simulink model "Smart_City_QCar2_VIRTUAL_car5_r2020a"  (R2020a)
settings: Solver=ode1  StartTime=0.0  StopTime=inf  FixedStep=Controller_Sample_Time  RelTol=1e-3  EnableMultiTasking=on
undefined symbols (not defined in the file): Audio_Sample_Time, cameraStepSize, CSI_Sample_Time, DiscIntNeverNeededParam, gcbh, ImageDisplay_Sample_Time, Initialization_Time, Joystick_Sample_Time, JPEG, LiDAR_Sample_Time, map_mask, NN_Sample_Time, path_x, path_x2, path_x3, path_x4, path_x5, path_x6, path_x7, path_y, path_y2, path_y3, path_y4, path_y5, path_y6, path_y7, qc_get_step_size, RealSense_Sample_Time, video_display_show
libraries: quarc_library x61, simulink_extras x9, simulink x5
(part 3 of 4)

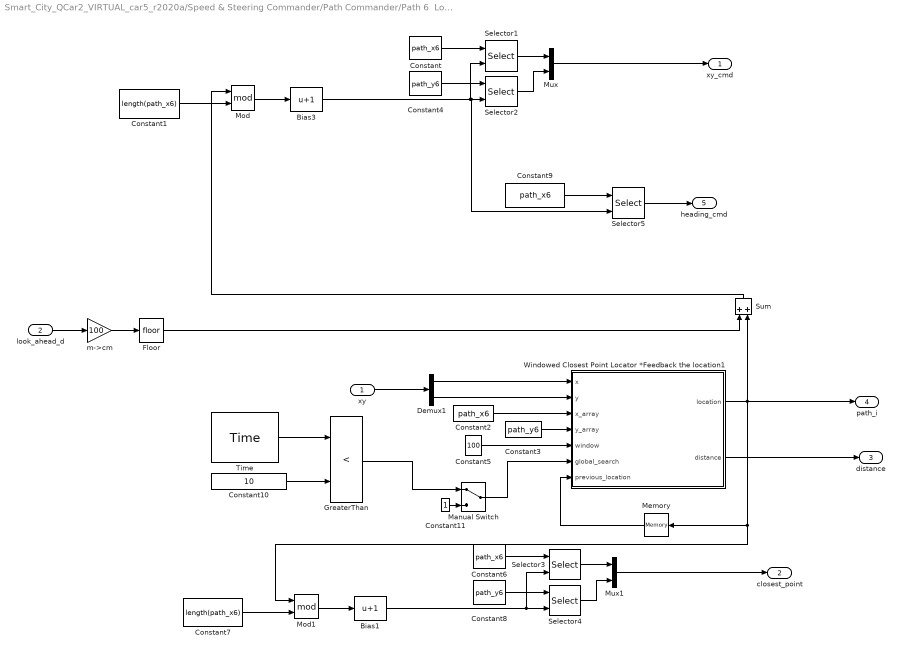
== system Smart_City_QCar2_VIRTUAL_car5_r2020a/Speed & Steering Commander/Path Commander/Path 6  Look Ahead Generator ==
  xy : Inport
  look_ahead_d : Inport  Port=2
  Bias1 : Bias  Bias=1
  Bias3 : Bias  Bias=1
  Constant{,2,6,9} (4 alike) : Constant  Value=path_x6
  Constant1 : Constant  Value=length(path_x6)
  Constant10 : Constant  Value=10
  Constant11 : Constant
  Constant3 : Constant  Value=path_y6
  Constant4 : Constant  Value=path_y6
  Constant5 : Constant  Value=100
  Constant7 : Constant  Value=length(path_x6)
  Constant8 : Constant  Value=path_y6
  Demux1 : Demux  Outputs=2
  Floor : Rounding
  GreaterThan : RelationalOperator  Operator=<  OutDataTypeStr=boolean  RndMeth=Simplest
  Manual Switch : ManualSwitch
  Memory : Memory  InitialCondition=1  InheritSampleTime=on  LinearizeMemory=on  LinearizeAsDelay=on
  Mod : Math  Operator=mod  SaturateOnIntegerOverflow=on
  Mod1 : Math  Operator=mod  SaturateOnIntegerOverflow=on
  Mux : Mux  Inputs=2
  Mux1 : Mux  Inputs=2
  Selector{1..5} (5 alike) : Selector  InputPortWidth=length(path_x6)  IndexOptions=Index vector (port)  Indices=[1 3]  OutputSizes=1
  Sum : Sum
  Time : quarc_library/Sources/Time/Time  time_source=Wall clock  sample_time=qc_get_step_size
  Windowed Closest Point Locator *Feedback the location1 : MATLAB Function  TreatAsAtomicUnit=on
  m->cm : Gain  Gain=100
  xy_cmd : Outport
  closest_point : Outport  Port=2
  distance : Outport  Port=3
  path_i : Outport  Port=4
  heading_cmd : Outport  Port=5
  wires:
  Windowed Closest Point Locator *Feedback the location1/1(location) -> Mod1/1, Memory/1, path_i/1, Sum/2
  Memory/1 -> Windowed Closest Point Locator *Feedback the location1/7(previous_location)
  Constant5/1 -> Windowed Closest Point Locator *Feedback the location1/5(window)
  Selector5/1 -> heading_cmd/1
  Constant9/1 -> Selector5/1
  Bias3/1 -> Selector2/2, Selector5/2, Selector1/2
  Windowed Closest Point Locator *Feedback the location1/2(distance) -> distance/1
  Selector2/1 -> Mux/2
  Mux/1 -> xy_cmd/1
  Constant4/1 -> Selector2/1
  Selector1/1 -> Mux/1
  Constant/1 -> Selector1/1
  Floor/1 -> Sum/1
  m->cm/1 -> Floor/1
  look_ahead_d/1 -> m->cm/1
  xy/1 -> Demux1/1
  Mod/1 -> Bias3/1
  Demux1/2 -> Windowed Closest Point Locator *Feedback the location1/2(y)
  Sum/1 -> Mod/1
  Constant1/1 -> Mod/2
  Constant3/1 -> Windowed Closest Point Locator *Feedback the location1/4(y_array)
  Constant2/1 -> Windowed Closest Point Locator *Feedback the location1/3(x_array)
  Demux1/1 -> Windowed Closest Point Locator *Feedback the location1/1(x)
  Mux1/1 -> closest_point/1
  Mod1/1 -> Bias1/1
  Selector4/1 -> Mux1/2
  Constant7/1 -> Mod1/2
  Selector3/1 -> Mux1/1
  Constant8/1 -> Selector4/1
  Bias1/1 -> Selector3/2, Selector4/2
  Constant6/1 -> Selector3/1
  Time/1 -> GreaterThan/1
  Constant10/1 -> GreaterThan/2
  Manual Switch/1 -> Windowed Closest Point Locator *Feedback the location1/6(global_search)
  Constant11/1 -> Manual Switch/2
  GreaterThan/1 -> Manual Switch/1

== system Smart_City_QCar2_VIRTUAL_car5_r2020a/Speed & Steering Commander/Path Commander/Path 7  Look Ahead Generator ==
  xy : Inport
  look_ahead_d : Inport  Port=2
  Bias1 : Bias  Bias=1
  Bias3 : Bias  Bias=1
  Constant{,2,6,9} (4 alike) : Constant  Value=path_x7
  Constant1 : Constant  Value=length(path_x7)
  Constant10 : Constant  Value=10
  Constant11 : Constant
  Constant3 : Constant  Value=path_y7
  Constant4 : Constant  Value=path_y7
  Constant5 : Constant  Value=100
  Constant7 : Constant  Value=length(path_x7)
  Constant8 : Constant  Value=path_y7
  Demux1 : Demux  Outputs=2
  Floor : Rounding
  GreaterThan : RelationalOperator  Operator=<  OutDataTypeStr=boolean  RndMeth=Simplest
  Manual Switch : ManualSwitch
  Memory : Memory  InitialCondition=1  InheritSampleTime=on  LinearizeMemory=on  LinearizeAsDelay=on
  Mod : Math  Operator=mod  SaturateOnIntegerOverflow=on
  Mod1 : Math  Operator=mod  SaturateOnIntegerOverflow=on
  Mux : Mux  Inputs=2
  Mux1 : Mux  Inputs=2
  Selector{1..5} (5 alike) : Selector  InputPortWidth=length(path_x7)  IndexOptions=Index vector (port)  Indices=[1 3]  OutputSizes=1
  Sum : Sum
  Time : quarc_library/Sources/Time/Time  time_source=Wall clock  sample_time=qc_get_step_size
  Windowed Closest Point Locator *Feedback the location1 : MATLAB Function  TreatAsAtomicUnit=on
  m->cm : Gain  Gain=100
  xy_cmd : Outport
  closest_point : Outport  Port=2
  distance : Outport  Port=3
  path_i : Outport  Port=4
  heading_cmd : Outport  Port=5
  wires:
  Windowed Closest Point Locator *Feedback the location1/1(location) -> Mod1/1, Memory/1, path_i/1, Sum/2
  Memory/1 -> Windowed Closest Point Locator *Feedback the location1/7(previous_location)
  Constant5/1 -> Windowed Closest Point Locator *Feedback the location1/5(window)
  Selector5/1 -> heading_cmd/1
  Constant9/1 -> Selector5/1
  Bias3/1 -> Selector2/2, Selector5/2, Selector1/2
  Windowed Closest Point Locator *Feedback the location1/2(distance) -> distance/1
  Selector2/1 -> Mux/2
  Mux/1 -> xy_cmd/1
  Constant4/1 -> Selector2/1
  Selector1/1 -> Mux/1
  Constant/1 -> Selector1/1
  Floor/1 -> Sum/1
  m->cm/1 -> Floor/1
  look_ahead_d/1 -> m->cm/1
  xy/1 -> Demux1/1
  Mod/1 -> Bias3/1
  Demux1/2 -> Windowed Closest Point Locator *Feedback the location1/2(y)
  Sum/1 -> Mod/1
  Constant1/1 -> Mod/2
  Constant3/1 -> Windowed Closest Point Locator *Feedback the location1/4(y_array)
  Constant2/1 -> Windowed Closest Point Locator *Feedback the location1/3(x_array)
  Demux1/1 -> Windowed Closest Point Locator *Feedback the location1/1(x)
  Mux1/1 -> closest_point/1
  Mod1/1 -> Bias1/1
  Selector4/1 -> Mux1/2
  Constant7/1 -> Mod1/2
  Selector3/1 -> Mux1/1
  Constant8/1 -> Selector4/1
  Bias1/1 -> Selector3/2, Selector4/2
  Constant6/1 -> Selector3/1
  Time/1 -> GreaterThan/1
  Constant10/1 -> GreaterThan/2
  Manual Switch/1 -> Windowed Closest Point Locator *Feedback the location1/6(global_search)
  Constant11/1 -> Manual Switch/2
  GreaterThan/1 -> Manual Switch/1

== system Smart_City_QCar2_VIRTUAL_car5_r2020a/Speed & Steering Commander/Steering Based on LiDAR/Direction Vector Generator ==
  xy_command : Inport
  xy : Inport  Port=2
  heading : Inport  Port=3
  Demux : Demux  Outputs=2
  Display2 : Display  Commented=on
      settings: Decimation=100
  Display5 : Display  Commented=on
      settings: Decimation=100
  Display8 : Display  Commented=on
      settings: Decimation=100
  Radians to Degrees1 : simulink_extras/Transformations/Radians to Degrees
  Radians to Degrees3 : simulink_extras/Transformations/Radians to Degrees
  Signed Sqrt : Sqrt  SaturateOnIntegerOverflow=on
  Square : Math  Operator=square  SaturateOnIntegerOverflow=on
  Sum : Sum  Inputs=+-
  Sum1 : Sum  Inputs=+
  Sum3 : Sum  Inputs=+-
  Trigonometric Function : Trigonometry  Operator=atan2
  distance : Outport
  aoa : Outport  Port=2
  wires:
  heading/1 -> Sum3/2
  Sum/1 -> Demux/1, Square/1
  Radians to Degrees3/1 -> Display2/1
  Radians to Degrees1/1 -> Display5/1
  Demux/2 -> Trigonometric Function/1
  Sum1/1 -> Signed Sqrt/1
  Sum3/1 -> aoa/1, Radians to Degrees3/1
  xy/1 -> Sum/2
  Signed Sqrt/1 -> distance/1, Display8/1
  Square/1 -> Sum1/1
  Trigonometric Function/1 -> Radians to Degrees1/1, Sum3/1
  Demux/1 -> Trigonometric Function/2
  xy_command/1 -> Sum/1

== system Smart_City_QCar2_VIRTUAL_car5_r2020a/Speed & Steering Commander/Traffic Zone 1/Greater Than Threshold ==
  Signal : Inport
  Threshold : Inport  Port=2
  Duration : Inport  Port=3
  Data Type Conversion : DataTypeConversion
  Discrete-Time Integrator : DiscreteIntegrator  Priority=1  ExternalReset=level  SampleTime=qc_get_step_size  ICPrevOutput=DiscIntNeverNeededParam  ICPrevScaledInput=DiscIntNeverNeededParam
  Logical Operator : Logic  Operator=NOT  AllPortsSameDT=off  OutDataTypeStr=boolean
  Relational Operator : RelationalOperator  RndMeth=Nearest
  Relational Operator1 : RelationalOperator  RndMeth=Nearest
  elapsed : Outport  VectorParamsAs1DForOutWhenUnconnected=off
  time : Outport  Port=2  VectorParamsAs1DForOutWhenUnconnected=off
  wires:
  Data Type Conversion/1 -> Discrete-Time Integrator/1
  Signal/1 -> Relational Operator/1
  Threshold/1 -> Relational Operator/2
  Relational Operator/1 -> Data Type Conversion/1, Logical Operator/1
  Logical Operator/1 -> Discrete-Time Integrator/2
  Discrete-Time Integrator/1 -> Relational Operator1/1, time/1
  Duration/1 -> Relational Operator1/2
  Relational Operator1/1 -> elapsed/1

== system Smart_City_QCar2_VIRTUAL_car5_r2020a/Speed & Steering Commander/Traffic Zone 1/Less Than Threshold ==
  Signal : Inport
  Threshold : Inport  Port=2
  Duration : Inport  Port=3
  Data Type Conversion : DataTypeConversion
  Discrete-Time Integrator : DiscreteIntegrator  Priority=1  ExternalReset=level  SampleTime=qc_get_step_size  ICPrevOutput=DiscIntNeverNeededParam  ICPrevScaledInput=DiscIntNeverNeededParam
  Logical Operator : Logic  Operator=NOT  AllPortsSameDT=off  OutDataTypeStr=boolean
  Relational Operator : RelationalOperator  Operator=<  RndMeth=Nearest
  Relational Operator1 : RelationalOperator  RndMeth=Nearest
  elapsed : Outport  VectorParamsAs1DForOutWhenUnconnected=off
  time : Outport  Port=2  VectorParamsAs1DForOutWhenUnconnected=off
  wires:
  Relational Operator1/1 -> elapsed/1
  Duration/1 -> Relational Operator1/2
  Discrete-Time Integrator/1 -> time/1, Relational Operator1/1
  Logical Operator/1 -> Discrete-Time Integrator/2
  Relational Operator/1 -> Logical Operator/1, Data Type Conversion/1
  Threshold/1 -> Relational Operator/2
  Signal/1 -> Relational Operator/1
  Data Type Conversion/1 -> Discrete-Time Integrator/1

== system Smart_City_QCar2_VIRTUAL_car5_r2020a/Speed & Steering Commander/Traffic Zone 2/Greater Than Threshold ==
  Signal : Inport
  Threshold : Inport  Port=2
  Duration : Inport  Port=3
  Data Type Conversion : DataTypeConversion
  Discrete-Time Integrator : DiscreteIntegrator  Priority=1  ExternalReset=level  SampleTime=qc_get_step_size  ICPrevOutput=DiscIntNeverNeededParam  ICPrevScaledInput=DiscIntNeverNeededParam
  Logical Operator : Logic  Operator=NOT  AllPortsSameDT=off  OutDataTypeStr=boolean
  Relational Operator : RelationalOperator  RndMeth=Nearest
  Relational Operator1 : RelationalOperator  RndMeth=Nearest
  elapsed : Outport  VectorParamsAs1DForOutWhenUnconnected=off
  time : Outport  Port=2  VectorParamsAs1DForOutWhenUnconnected=off
  wires:
  Relational Operator1/1 -> elapsed/1
  Duration/1 -> Relational Operator1/2
  Discrete-Time Integrator/1 -> time/1, Relational Operator1/1
  Logical Operator/1 -> Discrete-Time Integrator/2
  Relational Operator/1 -> Logical Operator/1, Data Type Conversion/1
  Threshold/1 -> Relational Operator/2
  Signal/1 -> Relational Operator/1
  Data Type Conversion/1 -> Discrete-Time Integrator/1

== system Smart_City_QCar2_VIRTUAL_car5_r2020a/Speed & Steering Commander/Traffic Zone 2/Less Than Threshold ==
  Signal : Inport
  Threshold : Inport  Port=2
  Duration : Inport  Port=3
  Data Type Conversion : DataTypeConversion
  Discrete-Time Integrator : DiscreteIntegrator  Priority=1  ExternalReset=level  SampleTime=qc_get_step_size  ICPrevOutput=DiscIntNeverNeededParam  ICPrevScaledInput=DiscIntNeverNeededParam
  Logical Operator : Logic  Operator=NOT  AllPortsSameDT=off  OutDataTypeStr=boolean
  Relational Operator : RelationalOperator  Operator=<  RndMeth=Nearest
  Relational Operator1 : RelationalOperator  RndMeth=Nearest
  elapsed : Outport  VectorParamsAs1DForOutWhenUnconnected=off
  time : Outport  Port=2  VectorParamsAs1DForOutWhenUnconnected=off
  wires:
  Data Type Conversion/1 -> Discrete-Time Integrator/1
  Signal/1 -> Relational Operator/1
  Threshold/1 -> Relational Operator/2
  Relational Operator/1 -> Data Type Conversion/1, Logical Operator/1
  Logical Operator/1 -> Discrete-Time Integrator/2
  Discrete-Time Integrator/1 -> Relational Operator1/1, time/1
  Duration/1 -> Relational Operator1/2
  Relational Operator1/1 -> elapsed/1

== system Smart_City_QCar2_VIRTUAL_car5_r2020a/QCar/Virtual QCar/LED Logic/Greater Than Threshold1 ==
  Signal : Inport
  Threshold : Inport  Port=2
  Duration : Inport  Port=3
  Data Type Conversion : DataTypeConversion
  Discrete-Time Integrator : DiscreteIntegrator  Priority=1  ExternalReset=level  SampleTime=qc_get_step_size  ICPrevOutput=DiscIntNeverNeededParam  ICPrevScaledInput=DiscIntNeverNeededParam
  Logical Operator : Logic  Operator=NOT  AllPortsSameDT=off  OutDataTypeStr=boolean
  Relational Operator : RelationalOperator  RndMeth=Nearest
  Relational Operator1 : RelationalOperator  RndMeth=Nearest
  elapsed : Outport  VectorParamsAs1DForOutWhenUnconnected=off
  time : Outport  Port=2  VectorParamsAs1DForOutWhenUnconnected=off
  wires:
  Data Type Conversion/1 -> Discrete-Time Integrator/1
  Signal/1 -> Relational Operator/1
  Threshold/1 -> Relational Operator/2
  Relational Operator/1 -> Data Type Conversion/1, Logical Operator/1
  Logical Operator/1 -> Discrete-Time Integrator/2
  Discrete-Time Integrator/1 -> Relational Operator1/1, time/1
  Duration/1 -> Relational Operator1/2
  Relational Operator1/1 -> elapsed/1

== system Smart_City_QCar2_VIRTUAL_car5_r2020a/QCar/Virtual QCar/LED Logic/Left Threshold ==
  Signal : Inport
  Threshold : Inport  Port=2
  Duration : Inport  Port=3
  Data Type Conversion : DataTypeConversion
  Discrete-Time Integrator : DiscreteIntegrator  Priority=1  ExternalReset=level  SampleTime=qc_get_step_size  ICPrevOutput=DiscIntNeverNeededParam  ICPrevScaledInput=DiscIntNeverNeededParam
  Logical Operator : Logic  Operator=NOT  AllPortsSameDT=off  OutDataTypeStr=boolean
  Relational Operator : RelationalOperator  RndMeth=Nearest
  Relational Operator1 : RelationalOperator  RndMeth=Nearest
  elapsed : Outport  VectorParamsAs1DForOutWhenUnconnected=off
  time : Outport  Port=2  VectorParamsAs1DForOutWhenUnconnected=off
  wires:
  Data Type Conversion/1 -> Discrete-Time Integrator/1
  Signal/1 -> Relational Operator/1
  Threshold/1 -> Relational Operator/2
  Relational Operator/1 -> Data Type Conversion/1, Logical Operator/1
  Logical Operator/1 -> Discrete-Time Integrator/2
  Discrete-Time Integrator/1 -> Relational Operator1/1, time/1
  Duration/1 -> Relational Operator1/2
  Relational Operator1/1 -> elapsed/1

== system Smart_City_QCar2_VIRTUAL_car5_r2020a/QCar/Virtual QCar/LED Logic/Less Than Threshold1 ==
  Signal : Inport
  Threshold : Inport  Port=2
  Duration : Inport  Port=3
  Data Type Conversion : DataTypeConversion
  Discrete-Time Integrator : DiscreteIntegrator  Priority=1  ExternalReset=level  SampleTime=qc_get_step_size  ICPrevOutput=DiscIntNeverNeededParam  ICPrevScaledInput=DiscIntNeverNeededParam
  Logical Operator : Logic  Operator=NOT  AllPortsSameDT=off  OutDataTypeStr=boolean
  Relational Operator : RelationalOperator  Operator=<  RndMeth=Nearest
  Relational Operator1 : RelationalOperator  RndMeth=Nearest
  elapsed : Outport  VectorParamsAs1DForOutWhenUnconnected=off
  time : Outport  Port=2  VectorParamsAs1DForOutWhenUnconnected=off
  wires:
  Relational Operator1/1 -> elapsed/1
  Duration/1 -> Relational Operator1/2
  Discrete-Time Integrator/1 -> time/1, Relational Operator1/1
  Logical Operator/1 -> Discrete-Time Integrator/2
  Relational Operator/1 -> Logical Operator/1, Data Type Conversion/1
  Threshold/1 -> Relational Operator/2
  Signal/1 -> Relational Operator/1
  Data Type Conversion/1 -> Discrete-Time Integrator/1

== system Smart_City_QCar2_VIRTUAL_car5_r2020a/QCar/Virtual QCar/LED Logic/Less Than Threshold2 ==
  Signal : Inport
  Threshold : Inport  Port=2
  Duration : Inport  Port=3
  Data Type Conversion : DataTypeConversion
  Discrete-Time Integrator : DiscreteIntegrator  Priority=1  ExternalReset=level  SampleTime=qc_get_step_size  ICPrevOutput=DiscIntNeverNeededParam  ICPrevScaledInput=DiscIntNeverNeededParam
  Logical Operator : Logic  Operator=NOT  AllPortsSameDT=off  OutDataTypeStr=boolean
  Relational Operator : RelationalOperator  Operator=<  RndMeth=Nearest
  Relational Operator1 : RelationalOperator  RndMeth=Nearest
  elapsed : Outport  VectorParamsAs1DForOutWhenUnconnected=off
  time : Outport  Port=2  VectorParamsAs1DForOutWhenUnconnected=off
  wires:
  Data Type Conversion/1 -> Discrete-Time Integrator/1
  Signal/1 -> Relational Operator/1
  Threshold/1 -> Relational Operator/2
  Relational Operator/1 -> Data Type Conversion/1, Logical Operator/1
  Logical Operator/1 -> Discrete-Time Integrator/2
  Discrete-Time Integrator/1 -> Relational Operator1/1, time/1
  Duration/1 -> Relational Operator1/2
  Relational Operator1/1 -> elapsed/1

== system Smart_City_QCar2_VIRTUAL_car5_r2020a/QCar/Virtual QCar/LED Logic/Less Than Threshold3 ==
  Signal : Inport
  Threshold : Inport  Port=2
  Duration : Inport  Port=3
  Data Type Conversion : DataTypeConversion
  Discrete-Time Integrator : DiscreteIntegrator  Priority=1  ExternalReset=level  SampleTime=qc_get_step_size  ICPrevOutput=DiscIntNeverNeededParam  ICPrevScaledInput=DiscIntNeverNeededParam
  Logical Operator : Logic  Operator=NOT  AllPortsSameDT=off  OutDataTypeStr=boolean
  Relational Operator : RelationalOperator  Operator=<  RndMeth=Nearest
  Relational Operator1 : RelationalOperator  RndMeth=Nearest
  elapsed : Outport  VectorParamsAs1DForOutWhenUnconnected=off
  time : Outport  Port=2  VectorParamsAs1DForOutWhenUnconnected=off
  wires:
  Relational Operator1/1 -> elapsed/1
  Duration/1 -> Relational Operator1/2
  Discrete-Time Integrator/1 -> time/1, Relational Operator1/1
  Logical Operator/1 -> Discrete-Time Integrator/2
  Relational Operator/1 -> Logical Operator/1, Data Type Conversion/1
  Threshold/1 -> Relational Operator/2
  Signal/1 -> Relational Operator/1
  Data Type Conversion/1 -> Discrete-Time Integrator/1

== system Smart_City_QCar2_VIRTUAL_car5_r2020a/QCar/Virtual QCar/LED Logic/Right Threshold ==
  Signal : Inport
  Threshold : Inport  Port=2
  Duration : Inport  Port=3
  Data Type Conversion : DataTypeConversion
  Discrete-Time Integrator : DiscreteIntegrator  Priority=1  ExternalReset=level  SampleTime=qc_get_step_size  ICPrevOutput=DiscIntNeverNeededParam  ICPrevScaledInput=DiscIntNeverNeededParam
  Logical Operator : Logic  Operator=NOT  AllPortsSameDT=off  OutDataTypeStr=boolean
  Relational Operator : RelationalOperator  Operator=<  RndMeth=Nearest
  Relational Operator1 : RelationalOperator  RndMeth=Nearest
  elapsed : Outport  VectorParamsAs1DForOutWhenUnconnected=off
  time : Outport  Port=2  VectorParamsAs1DForOutWhenUnconnected=off
  wires:
  Data Type Conversion/1 -> Discrete-Time Integrator/1
  Signal/1 -> Relational Operator/1
  Threshold/1 -> Relational Operator/2
  Relational Operator/1 -> Data Type Conversion/1, Logical Operator/1
  Logical Operator/1 -> Discrete-Time Integrator/2
  Discrete-Time Integrator/1 -> Relational Operator1/1, time/1
  Duration/1 -> Relational Operator1/2
  Relational Operator1/1 -> elapsed/1

== matlab function Smart_City_QCar2_VIRTUAL_car5_r2020a/Speed & Steering Commander/Infrastructure Car Detection Speed Adjust/MATLAB Function ==
  data: obstacle_distance input; speed_cmd output; stop_distance input; nominal_tracking_distance input; nominal_speed input
function speed_cmd = adaptive_cruise_control(obstacle_distance, stop_distance, nominal_tracking_distance, nominal_speed)

speed_cmd = nominal_speed;

if obstacle_distance < stop_distance
    speed_cmd = sat(nominal_speed,0,-1);
    
elseif obstacle_distance < nominal_tracking_distance
    speed_cmd = nominal_speed/(nominal_tracking_distance-stop_distance)*obstacle_distance...
        - nominal_speed/(nominal_tracking_distance-stop_distance)*stop_distance;
    
end

function output = sat (input, max,min)
if input > max
    output = max;
elseif input < min
    output = min;
else
    output = input;
end

== matlab function Smart_City_QCar2_VIRTUAL_car5_r2020a/Speed & Steering Commander/Traffic Zone 2/MATLAB Function2 ==
  data: Previous_State input; Speed_In input; Speed_Multi input; In_Zone input; Traffic_State output; Speed_Out output; Traffic_Light input
function [Traffic_State, Speed_Out]  = Traffic_Controller (Previous_State, Speed_In, Speed_Multi, In_Zone, Traffic_Light)
%#codegen
Traffic_State = Previous_State;
Speed_Out = Speed_In;

switch Traffic_State
    % Case 1 - Normal - either not in zone or green light, Case 2 - red
    % light and in zone
    
    case 1
        % Green light or not in zone
        Speed_Out = Speed_In;
        if (Traffic_Light == 0) && (In_Zone == 1)
            % Caught in the traffic controller's web!
            Traffic_State = 2;
        end
        
    case 2
        % Red light state
        Speed_Out = Speed_In * Speed_Multi;
        
        if (Traffic_Light == 1)
            % Green Light
            Traffic_State = 1;
        end
        
end
end

== matlab function Smart_City_QCar2_VIRTUAL_car5_r2020a/QCar/To//From Simulation/Receive Fcn ==
  data: Receive input size=800000; RequestServerUpdate output; New input; Location output; Rotation output; BumpForward output; BumpRear output; EnvironmentReset output; LidarDist output; LidarAngle output; NewCSIRight output; ImageCSIRight output size=100000; NewCSIRear output; ImageCSIRear output size=100000; NewCSILeft output; ImageCSILeft output size=100000; NewCSIFront output; ImageCSIFront output size=100000; NewRGB output; ImageRGB output size=100000; NewDepth output; ImageDepth output size=100000; Debug output
function [RequestServerUpdate, Location, Rotation, BumpForward, BumpRear, EnvironmentReset, LidarDist, LidarAngle, ...
    NewCSIRight, ImageCSIRight, ...
    NewCSIRear, ImageCSIRear, ...
    NewCSILeft, ImageCSILeft, ...
    NewCSIFront, ImageCSIFront, ...
    NewRGB, ImageRGB, ...
    NewDepth, ImageDepth, ...
    Debug]  = QCar2ApplicationWorkspaceDecodeDataPacket(Receive, New)

%% Setup

LIDAR_SAMPLES = 384;
LIDAR_RANGE = 80;

persistent iLocation;
persistent iRotation;
persistent iBumpForward;
persistent iBumpRear;
persistent iLidarDist;
persistent iLidarAngle;

if isempty(iLocation)
    iLocation = [single(0); single(0); single(0)];
    iRotation = [single(0); single(0); single(0)];
    iBumpForward = uint8(0);
    iBumpRear = uint8(0);
    iLidarAngle = zeros(1,LIDAR_SAMPLES);   
    iLidarDist = zeros(1,LIDAR_SAMPLES);      
end

% Need to assign outputs here even though they are reassigned at the end
% since matlab can't determine the signal widths
Location = [single(0); single(0); single(0)];
Rotation = [single(0); single(0); single(0)];
BumpForward = uint8(0);
BumpRear = uint8(0);
EnvironmentReset = 0;

LidarAngle = zeros(1,LIDAR_SAMPLES);
LidarDist = zeros(1,LIDAR_SAMPLES);

ImageCSIRight = uint8([]);
NewCSIRight = 0;
ImageCSIRear = uint8([]);
NewCSIRear = 0;
ImageCSILeft = uint8([]);
NewCSILeft = 0;
ImageCSIFront = uint8([]);
NewCSIFront = 0;
ImageRGB = uint8([]);
NewRGB = 0;
ImageDepth = uint8([]);
NewDepth = 0;


RequestServerUpdate = uint8(0);
PacketSize = length(Receive);

Debug = int32(0);

% Packet > 0, new data, and magic number in first index
if ((PacketSize > 0) && (New == 1) && (Receive(1) == uint8(123)))
    
    %skip magic number
    Index = int32(2);
    
    while(Index <= PacketSize)
       
        %% Get container details
        ContainerSize = typecast(uint8(flip(Receive(Index:Index+3))), 'int32');
        DeviceID = typecast(uint8(flip(Receive(Index+4:Index+7))), 'int32');
        DeviceNum = typecast(uint8(flip(Receive(Index+8:Index+11))), 'int32');
        DeviceFunction = uint8(Receive(Index+12));
        PayloadStart = Index+13;
        PayloadEnd = Index+ContainerSize-1;
        
        %% Pass container to appropriate decoding function
        if (DeviceID == 161) %is this a QCar 2 container?
            
            if (DeviceFunction == 11) %UE4 State Response
                [iLocation, iRotation, iBumpForward, iBumpRear] = QCar2DecodeVelocityStateContainer(Receive, PayloadStart);
                RequestServerUpdate = uint8(11);
            elseif (DeviceFunction == 101) % Pull out RGB payload for external processing
                CameraNum = typecast(uint8(flip(Receive(PayloadStart:PayloadStart+3))), 'int32');
                ImageSize = typecast(uint8(flip(Receive(PayloadStart+4:PayloadStart+7))), 'int32');
                
                if CameraNum == 0
                    ImageCSIRight = Receive(PayloadStart+8:PayloadEnd);
                    NewCSIRight = 1;
                    
                elseif CameraNum == 1
                    ImageCSIRear = Receive(PayloadStart+8:PayloadEnd);
                    NewCSIRear = 1;
                    
                elseif CameraNum == 2
                    ImageCSILeft = Receive(PayloadStart+8:PayloadEnd);
                    NewCSILeft = 1;
                    
                elseif CameraNum == 3
                    ImageCSIFront = Receive(PayloadStart+8:PayloadEnd);
                    NewCSIFront = 1;
                    
                elseif CameraNum == 4
                    ImageRGB = Receive(PayloadStart+8:PayloadEnd);
                    NewRGB = 1;
                    
                elseif CameraNum == 5
                    ImageDepth = Receive(PayloadStart+8:PayloadEnd);
                    NewDepth = 1;
                end
                RequestServerUpdate = uint8(1);

            elseif (DeviceFunction == 111) % Process LIDAR
                [iLidarAngle, iLidarDist] = QCar2DecodeLidarContainer(Receive, PayloadStart, LIDAR_SAMPLES, LIDAR_RANGE);
                RequestServerUpdate = uint8(1);                
            end
        elseif (DeviceID == 1001) %Simulink notification
            if (DeviceFunction == 200) %Reset button
                EnvironmentReset = 1;
            end
            


        end
       
        
        %% Process next container if any data is left.
        Index = Index+ContainerSize;
    end


end

Location = iLocation;
Rotation = iRotation;
BumpForward = iBumpForward;
BumpRear = iBumpRear;
LidarDist = iLidarDist;
LidarAngle = iLidarAngle;

== matlab function Smart_City_QCar2_VIRTUAL_car5_r2020a/Speed & Steering Commander/Realsense Obstacle Detection Speed Adjust/MATLAB Function ==
  data: obstacle_distance input; speed_cmd output; stop_distance input; nominal_tracking_distance input; nominal_speed input
function speed_cmd = adaptive_cruise_control(obstacle_distance, stop_distance, nominal_tracking_distance, nominal_speed)

speed_cmd = nominal_speed;

if obstacle_distance < stop_distance
    speed_cmd = sat(nominal_speed,0,-1);
    
elseif obstacle_distance < nominal_tracking_distance
    speed_cmd = nominal_speed/(nominal_tracking_distance-stop_distance)*obstacle_distance...
        - nominal_speed/(nominal_tracking_distance-stop_distance)*stop_distance;
    
end

function output = sat (input, max,min)
if input > max
    output = max;
elseif input < min
    output = min;
else
    output = input;
end

== matlab function Smart_City_QCar2_VIRTUAL_car5_r2020a/QCar/Virtual QCar/LED Logic/MATLAB Function ==
  data: headlights input; lights output; breaklights input; reverseLights input; leftTurn input; rightTurn input; pulse input
function lights = fcn (headlights, breaklights, reverseLights, leftTurn, rightTurn, pulse)

lights = zeros(1,16);
brakes = zeros(1,4); %4
head = zeros(1,6);%6
left = zeros(1,2);%2
right = zeros(1,2);%2
reverse = zeros(1,2);%2

if breaklights
    brakes = ones(1,4);
end

if headlights
    head = ones(1,6);
end

if reverseLights
    reverse = ones(1,2);
end

if leftTurn
    left = ones(1,2);
end

if rightTurn
    right = ones(1,2);
end

right = right & pulse;
left = left & pulse;

lights(1:4) = brakes;
lights(5:6) = reverse;
lights(7) = left(1);
lights(8) = right(1);
lights(9:14) = head;
lights(15) = left(2);
lights(16) = right(2);

== matlab function Smart_City_QCar2_VIRTUAL_car5_r2020a/Speed & Steering Commander/Steering Based on LiDAR/Steering Commander ==
  data: steering output; aoa input
function steering  = steering_command(aoa)
steering = aoa;
if aoa < -pi
    steering = aoa+2*pi;
elseif aoa > pi
    steering = aoa-2*pi;
else
    steering = aoa;
end
end

== matlab function Smart_City_QCar2_VIRTUAL_car5_r2020a/Speed & Steering Commander/Path Commander/Path 7  Look Ahead Generator/Windowed Closest Point Locator *Feedback the location1 ==
  data: x input; location output; y input; x_array input; y_array input; window input; global_search input; distance output; previous_location input
function [location,distance] = find_closest_window_point(x,y,x_array,y_array, window, global_search, previous_location)
distance = 1e6;
location = previous_location;
array_length = length (x_array);

if (global_search == 1)
    
    %Search the whole array (usually at startup)
    for i =1:array_length
        d = (x-x_array(i))^2 + (y-y_array(i))^2;
        if d < distance
            distance = d;
            location = i;
        end
    end
    
else
    
    if (location + window) > array_length
        %We need to wrap from the end
        % loop one - end of array:
        for i = (location-window):array_length
            d = (x-x_array(i))^2 + (y-y_array(i))^2;
            if d < distance
                distance = d;
                location = i;
            end
        end
        % loop two - start of array:
        for i = 1:(location+window-array_length)
            d = (x-x_array(i))^2 + (y-y_array(i))^2;
            if d < distance
                distance = d;
                location = i;
            end
        end
        
    elseif (location-window) < 1
        %We need to wrap from the beginning
        % loop one - end of array:
        for i = (array_length+location-window):array_length
            d = (x-x_array(i))^2 + (y-y_array(i))^2;
            if d < distance
                distance = d;
                location = i;
            end
        end
        % loop two - start of array:
        for i = 1:(location+window)
            d = (x-x_array(i))^2 + (y-y_array(i))^2;
            if d < distance
                distance = d;
                location = i;
            end
        end
        
    else
        %no need to wrap
        for i = (location-window):(location+window)
            d = (x-x_array(i))^2 + (y-y_array(i))^2;
            if d < distance
                distance = d;
                location = i;
            end
        end
    end
    
end
distance = sqrt(distance);
end

== matlab function Smart_City_QCar2_VIRTUAL_car5_r2020a/RealSense Camera/obstacleDetection Markham March 22/Draw Lines Module ==
  data: img_in input; img_out output size=[480,640,3]; pts input; color input
function img_out = drawLines(img_in, pts, color)

% Draw lines connecting the points using the provided color

% Inputs:
% u         : Input RGB Image (size = m by n)
% pts       : p x-y pairs of points (px) where markers are to be drawn
% color     : 1x3 matrix of RGB color values for each marker

% Outputs:
% y         : Output RGB Image with the markers drawn in (size = m by n)

%% Initialization
img_out = cat(3, img_in, img_in, img_in);

[p, ~] = size(pts); % determine the number of points

%% Draw the lines
    for i = 1:p-1
        % determine the max(rows_difference, col_difference) between two
        % points
        itr = max(abs(pts(i,1) - pts(i+1,1)), abs(pts(i,2) - pts(i+1,2)));
        
        % generate linear spaces of row and col values between the pts
        row_vec = round(linspace(pts(i,1), pts(i+1,1), itr));
        col_vec = round(linspace(pts(i,2), pts(i+1,2), itr));
        
        % iterate through the values and shade them right

        for j = 1:itr
            img_out(row_vec(j), col_vec(j),1) = color(1);
            img_out(row_vec(j), col_vec(j),2) = color(2);
            img_out(row_vec(j), col_vec(j),3) = color(3);
        end
    end
end

== matlab function Smart_City_QCar2_VIRTUAL_car5_r2020a/Speed & Steering Commander/Path Commander/Path 1  Look Ahead Generator/Windowed Closest Point Locator *Feedback the location1 ==
  data: x input; location output; y input; x_array input; y_array input; window input; global_search input; distance output; previous_location input
function [location,distance] = find_closest_window_point(x,y,x_array,y_array, window, global_search, previous_location)
distance = 1e6;
location = previous_location;
array_length = length (x_array);

if (global_search == 1)
    
    %Search the whole array (usually at startup)
    for i =1:array_length
        d = (x-x_array(i))^2 + (y-y_array(i))^2;
        if d < distance
            distance = d;
            location = i;
        end
    end
    
else
    
    if (location + window) > array_length
        %We need to wrap from the end
        % loop one - end of array:
        for i = (location-window):array_length
            d = (x-x_array(i))^2 + (y-y_array(i))^2;
            if d < distance
                distance = d;
                location = i;
            end
        end
        % loop two - start of array:
        for i = 1:(location+window-array_length)
            d = (x-x_array(i))^2 + (y-y_array(i))^2;
            if d < distance
                distance = d;
                location = i;
            end
        end
        
    elseif (location-window) < 1
        %We need to wrap from the beginning
        % loop one - end of array:
        for i = (array_length+location-window):array_length
            d = (x-x_array(i))^2 + (y-y_array(i))^2;
            if d < distance
                distance = d;
                location = i;
            end
        end
        % loop two - start of array:
        for i = 1:(location+window)
            d = (x-x_array(i))^2 + (y-y_array(i))^2;
            if d < distance
                distance = d;
                location = i;
            end
        end
        
    else
        %no need to wrap
        for i = (location-window):(location+window)
            d = (x-x_array(i))^2 + (y-y_array(i))^2;
            if d < distance
                distance = d;
                location = i;
            end
        end
    end
    
end
distance = sqrt(distance);
end

== matlab function Smart_City_QCar2_VIRTUAL_car5_r2020a/Speed & Steering Commander/Path Commander/Path 2  Look Ahead Generator/Windowed Closest Point Locator *Feedback the location1 ==
  data: x input; location output; y input; x_array input; y_array input; window input; global_search input; distance output; previous_location input
function [location,distance] = find_closest_window_point(x,y,x_array,y_array, window, global_search, previous_location)
distance = 1e6;
location = previous_location;
array_length = length (x_array);

if (global_search == 1)
    
    %Search the whole array (usually at startup)
    for i =1:array_length
        d = (x-x_array(i))^2 + (y-y_array(i))^2;
        if d < distance
            distance = d;
            location = i;
        end
    end
    
else
    
    if (location + window) > array_length
        %We need to wrap from the end
        % loop one - end of array:
        for i = (location-window):array_length
            d = (x-x_array(i))^2 + (y-y_array(i))^2;
            if d < distance
                distance = d;
                location = i;
            end
        end
        % loop two - start of array:
        for i = 1:(location+window-array_length)
            d = (x-x_array(i))^2 + (y-y_array(i))^2;
            if d < distance
                distance = d;
                location = i;
            end
        end
        
    elseif (location-window) < 1
        %We need to wrap from the beginning
        % loop one - end of array:
        for i = (array_length+location-window):array_length
            d = (x-x_array(i))^2 + (y-y_array(i))^2;
            if d < distance
                distance = d;
                location = i;
            end
        end
        % loop two - start of array:
        for i = 1:(location+window)
            d = (x-x_array(i))^2 + (y-y_array(i))^2;
            if d < distance
                distance = d;
                location = i;
            end
        end
        
    else
        %no need to wrap
        for i = (location-window):(location+window)
            d = (x-x_array(i))^2 + (y-y_array(i))^2;
            if d < distance
                distance = d;
                location = i;
            end
        end
    end
    
end
distance = sqrt(distance);
end

== matlab function Smart_City_QCar2_VIRTUAL_car5_r2020a/Speed & Steering Commander/Path Commander/Path 4  Look Ahead Generator/Windowed Closest Point Locator *Feedback the location1 ==
  data: x input; location output; y input; x_array input; y_array input; window input; global_search input; distance output; previous_location input
function [location,distance] = find_closest_window_point(x,y,x_array,y_array, window, global_search, previous_location)
distance = 1e6;
location = previous_location;
array_length = length (x_array);

if (global_search == 1)
    
    %Search the whole array (usually at startup)
    for i =1:array_length
        d = (x-x_array(i))^2 + (y-y_array(i))^2;
        if d < distance
            distance = d;
            location = i;
        end
    end
    
else
    
    if (location + window) > array_length
        %We need to wrap from the end
        % loop one - end of array:
        for i = (location-window):array_length
            d = (x-x_array(i))^2 + (y-y_array(i))^2;
            if d < distance
                distance = d;
                location = i;
            end
        end
        % loop two - start of array:
        for i = 1:(location+window-array_length)
            d = (x-x_array(i))^2 + (y-y_array(i))^2;
            if d < distance
                distance = d;
                location = i;
            end
        end
        
    elseif (location-window) < 1
        %We need to wrap from the beginning
        % loop one - end of array:
        for i = (array_length+location-window):array_length
            d = (x-x_array(i))^2 + (y-y_array(i))^2;
            if d < distance
                distance = d;
                location = i;
            end
        end
        % loop two - start of array:
        for i = 1:(location+window)
            d = (x-x_array(i))^2 + (y-y_array(i))^2;
            if d < distance
                distance = d;
                location = i;
            end
        end
        
    else
        %no need to wrap
        for i = (location-window):(location+window)
            d = (x-x_array(i))^2 + (y-y_array(i))^2;
            if d < distance
                distance = d;
                location = i;
            end
        end
    end
    
end
distance = sqrt(distance);
end

== matlab function Smart_City_QCar2_VIRTUAL_car5_r2020a/Speed & Steering Commander/Path Commander/Path 5  Look Ahead Generator/Windowed Closest Point Locator *Feedback the location1 ==
  data: x input; location output; y input; x_array input; y_array input; window input; global_search input; distance output; previous_location input
function [location,distance] = find_closest_window_point(x,y,x_array,y_array, window, global_search, previous_location)
distance = 1e6;
location = previous_location;
array_length = length (x_array);

if (global_search == 1)
    
    %Search the whole array (usually at startup)
    for i =1:array_length
        d = (x-x_array(i))^2 + (y-y_array(i))^2;
        if d < distance
            distance = d;
            location = i;
        end
    end
    
else
    
    if (location + window) > array_length
        %We need to wrap from the end
        % loop one - end of array:
        for i = (location-window):array_length
            d = (x-x_array(i))^2 + (y-y_array(i))^2;
            if d < distance
                distance = d;
                location = i;
            end
        end
        % loop two - start of array:
        for i = 1:(location+window-array_length)
            d = (x-x_array(i))^2 + (y-y_array(i))^2;
            if d < distance
                distance = d;
                location = i;
            end
        end
        
    elseif (location-window) < 1
        %We need to wrap from the beginning
        % loop one - end of array:
        for i = (array_length+location-window):array_length
            d = (x-x_array(i))^2 + (y-y_array(i))^2;
            if d < distance
                distance = d;
                location = i;
            end
        end
        % loop two - start of array:
        for i = 1:(location+window)
            d = (x-x_array(i))^2 + (y-y_array(i))^2;
            if d < distance
                distance = d;
                location = i;
            end
        end
        
    else
        %no need to wrap
        for i = (location-window):(location+window)
            d = (x-x_array(i))^2 + (y-y_array(i))^2;
            if d < distance
                distance = d;
                location = i;
            end
        end
    end
    
end
distance = sqrt(distance);
end

== matlab function Smart_City_QCar2_VIRTUAL_car5_r2020a/Speed & Steering Commander/Path Commander/Path 6  Look Ahead Generator/Windowed Closest Point Locator *Feedback the location1 ==
  data: x input; location output; y input; x_array input; y_array input; window input; global_search input; distance output; previous_location input
function [location,distance] = find_closest_window_point(x,y,x_array,y_array, window, global_search, previous_location)
distance = 1e6;
location = previous_location;
array_length = length (x_array);

if (global_search == 1)
    
    %Search the whole array (usually at startup)
    for i =1:array_length
        d = (x-x_array(i))^2 + (y-y_array(i))^2;
        if d < distance
            distance = d;
            location = i;
        end
    end
    
else
    
    if (location + window) > array_length
        %We need to wrap from the end
        % loop one - end of array:
        for i = (location-window):array_length
            d = (x-x_array(i))^2 + (y-y_array(i))^2;
            if d < distance
                distance = d;
                location = i;
            end
        end
        % loop two - start of array:
        for i = 1:(location+window-array_length)
            d = (x-x_array(i))^2 + (y-y_array(i))^2;
            if d < distance
                distance = d;
                location = i;
            end
        end
        
    elseif (location-window) < 1
        %We need to wrap from the beginning
        % loop one - end of array:
        for i = (array_length+location-window):array_length
            d = (x-x_array(i))^2 + (y-y_array(i))^2;
            if d < distance
                distance = d;
                location = i;
            end
        end
        % loop two - start of array:
        for i = 1:(location+window)
            d = (x-x_array(i))^2 + (y-y_array(i))^2;
            if d < distance
                distance = d;
                location = i;
            end
        end
        
    else
        %no need to wrap
        for i = (location-window):(location+window)
            d = (x-x_array(i))^2 + (y-y_array(i))^2;
            if d < distance
                distance = d;
                location = i;
            end
        end
    end
    
end
distance = sqrt(distance);
end

== matlab function Smart_City_QCar2_VIRTUAL_car5_r2020a/Infrastructure/Find Closest Car/MATLAB Function ==
  data: x_car input; distance output; y_car input; x_vector input; y_vector input; car_index input; heading input; proximity_radius input; proximity_scan_window input; max_distance input; distance_vector output; heading_vector output
function [distance, distance_vector, heading_vector] = proximity_sensor (x_car, y_car, x_vector, y_vector, car_index, heading, proximity_radius, proximity_scan_window, max_distance)
distance = max_distance;
distance_vector = max_distance + 0*x_vector;
heading_vector = 2*pi +  0*x_vector;

for i = 1:length (x_vector)
    if (i ~= car_index)
        distance_vector(i) = sqrt ((x_car - x_vector(i))^2 + (y_car - y_vector(i))^2);
        heading_vector(i) = atan2( (y_vector(i) - y_car), (x_vector(i) - x_car)) - heading;
        if (heading_vector(i) > pi)
            heading_vector(i) = heading_vector(i) - 2*pi;
        elseif (heading_vector(i) < -pi)
            heading_vector(i) = heading_vector(i) + 2*pi;
        end
        if ((distance_vector(i) < distance) && (abs (heading_vector(i)) <= proximity_scan_window))
            distance =  distance_vector(i);
        end
       
    end
end

== matlab function Smart_City_QCar2_VIRTUAL_car5_r2020a/Infrastructure/Find Closest Car/MATLAB Function1 ==
  data: speed input; proximity_scan_window output; max_speed input; min_window input; max_window input
function proximity_scan_window = scan_window_generator(speed, max_speed, min_window, max_window)
%#codegen
proximity_scan_window = min_window + speed*(max_window - min_window) / max_speed;
end

== matlab function Smart_City_QCar2_VIRTUAL_car5_r2020a/Speed & Steering Commander/Traffic Zone 1/MATLAB Function2 ==
  data: Previous_State input; Speed_In input; Speed_Multi input; In_Zone input; Traffic_State output; Speed_Out output; Traffic_Light input
function [Traffic_State, Speed_Out]  = Traffic_Controller (Previous_State, Speed_In, Speed_Multi, In_Zone, Traffic_Light)
%#codegen
Traffic_State = Previous_State;
Speed_Out = Speed_In;

switch Traffic_State
    % Case 1 - Normal - either not in zone or green light, Case 2 - red
    % light and in zone
    
    case 1
        % Green light or not in zone
        Speed_Out = Speed_In;
        if (Traffic_Light == 0) && (In_Zone == 1)
            % Caught in the traffic controller's web!
            Traffic_State = 2;
        end
        
    case 2
        % Red light state
        Speed_Out = Speed_In * Speed_Multi;
        
        if (Traffic_Light == 1)
            % Green Light
            Traffic_State = 1;
        end
        
end
end

== matlab function Smart_City_QCar2_VIRTUAL_car5_r2020a/RealSense Camera/obstacleDetection Markham March 22/Steering based image subselector ==
  data: pts output; depth input; distance output; steering input; minDistance input; maxDistance input; width input; height input; vertCenter input; maxSteering input; reduction input; maxSteeringWidth input; median_pts output; mean_pts output; min_pts output; max_pts output; num_pts output; pt_25 output; mean_middle output
function [pts, distance, median_pts, mean_pts, min_pts, max_pts, num_pts, pt_25, mean_middle] = estimateDepthInRegion(depth, steering, minDistance, maxDistance, width, height, vertCenter, maxSteering, reduction, maxSteeringWidth)
% Input: 640 x 480
[ROW, COL] = size(depth);
mark = COL/2 - (steering*(COL/2 - width/2)/maxSteering);
applied_width = max(width - abs(steering/maxSteeringWidth)*reduction*width, 60);
left_w = max(mark+1-(applied_width/2), 0); % pick the left end, but never let it get negative
right_w = min(left_w + applied_width, COL); % pick the right end, but never past the image width
upper_h = max(ROW*vertCenter-height/2+1, 0); % pick the upper end, but never let it get negative
lower_h = min(ROW*vertCenter+height/2, ROW); % pick the lower end, but never let it go past the image height
depth(:,1:40) = maxDistance; %this is to remove artifacts in the camera's left section
region = double(depth(upper_h:lower_h, left_w:right_w)); 
pts = [upper_h, left_w; upper_h, right_w; lower_h, right_w; lower_h, left_w; upper_h, left_w];

% reshape region of interest into 1D array
u_flat = reshape(region, 1, []);
% store a temp comparison matrix the size of u_flat
temp = maxDistance*ones(1, length(u_flat));

% compare u_flat to min and max distance
for i = 1:length(u_flat)
    % if u_flat is between min and max distance, store in temp array
    if (u_flat(i) >= minDistance) && (u_flat(i) <= maxDistance)
        temp(i) = u_flat(i);
    end
end

% u_flat(u_flat < minDistance) = [];
% u_flat(u_flat > maxDistance) = [];
% distance = mean(mean(u_flat));
distance = min(temp(:));
num_pts = 0;
median_pts = 0;
min_pts = 0;
mean_pts = 0;
max_pts = 0;

num_pts = length(temp);
median_pts = median (temp);
min_pts = min (temp);
max_pts = max (temp);
mean_pts = mean (temp);

% sort temp array small to large
sorted_points = sort (temp);
% pt_25 = 25% smallest distance in the array
pt_25 = sorted_points (floor(num_pts/4));
smaller_points = sorted_points (floor(num_pts/4):floor(num_pts*3/4));
mean_middle = mean (smaller_points);
